simulink model "ALU_Project"  (R2023b)
settings: Solver=VariableStepAuto  StartTime=0.0  StopTime=1  RelTol=1e-3
values from neighbouring files (symbols this model uses):
  A0 = str2num(get(handles.a0i,'string'))    [AluGui.m]
  A1 = str2num(get(handles.a1i,'string'))    [AluGui.m]
  A2 = str2num(get(handles.a2i,'string'))    [AluGui.m]
  A3 = str2num(get(handles.a3i,'string'))    [AluGui.m]
  B0 = str2num(get(handles.b0i,'string'))    [AluGui.m]
  B1 = str2num(get(handles.b1i,'string'))    [AluGui.m]
  B2 = str2num(get(handles.b2i,'string'))    [AluGui.m]
  B3 = str2num(get(handles.b3i,'string'))    [AluGui.m]
  Cin = str2num(get(handles.cii,'string'))    [AluGui.m]
undefined symbols (not defined in the file or in its folder): S0, S1, S2, S3
(part 2 of 2)

== system ALU_Project/15-DECREMENT/HAilf Adder 1 ==
  In1 : Inport
  In2 : Inport  Port=2
  AND : Logic  IconShape=distinctive  AllPortsSameDT=off  OutDataTypeStr=boolean
  XOR : Logic  Operator=XOR  IconShape=distinctive  AllPortsSameDT=off  OutDataTypeStr=boolean
  Sum : Outport
  Carry : Outport  Port=2
  wires:
  In1/1 -> AND/2, XOR/1
  XOR/1 -> Sum/1
  In2/1 -> XOR/2, AND/1
  AND/1 -> Carry/1

== system ALU_Project/15-DECREMENT/HAilf Adder 2 ==
  A1 : Inport
  In2 : Inport  Port=2
  AND : Logic  IconShape=distinctive  AllPortsSameDT=off  OutDataTypeStr=boolean
  XOR : Logic  Operator=XOR  IconShape=distinctive  AllPortsSameDT=off  OutDataTypeStr=boolean
  Sum : Outport
  Carry : Outport  Port=2
  wires:
  A1/1 -> AND/2, XOR/1
  XOR/1 -> Sum/1
  In2/1 -> XOR/2, AND/1
  AND/1 -> Carry/1

== system ALU_Project/15-DECREMENT/HAilf Adder 3 ==
  A2 : Inport
  In2 : Inport  Port=2
  AND : Logic  IconShape=distinctive  AllPortsSameDT=off  OutDataTypeStr=boolean
  XOR : Logic  Operator=XOR  IconShape=distinctive  AllPortsSameDT=off  OutDataTypeStr=boolean
  Sum : Outport
  Carry : Outport  Port=2
  wires:
  A2/1 -> AND/2, XOR/1
  XOR/1 -> Sum/1
  In2/1 -> XOR/2, AND/1
  AND/1 -> Carry/1

== system ALU_Project/15-DECREMENT/HAilf Adder 4 ==
  A3 : Inport
  In2 : Inport  Port=2
  AND : Logic  IconShape=distinctive  AllPortsSameDT=off  OutDataTypeStr=boolean
  XOR : Logic  Operator=XOR  IconShape=distinctive  AllPortsSameDT=off  OutDataTypeStr=boolean
  Sum : Outport
  Carry : Outport  Port=2
  wires:
  A3/1 -> AND/2, XOR/1
  XOR/1 -> Sum/1
  In2/1 -> XOR/2, AND/1
  AND/1 -> Carry/1

== system ALU_Project/15-DECREMENT/HAilf Adder 5 ==
  B0 : Inport
  In2 : Inport  Port=2
  AND : Logic  IconShape=distinctive  AllPortsSameDT=off  OutDataTypeStr=boolean
  XOR : Logic  Operator=XOR  IconShape=distinctive  AllPortsSameDT=off  OutDataTypeStr=boolean
  Sum : Outport
  Carry : Outport  Port=2
  wires:
  B0/1 -> AND/2, XOR/1
  XOR/1 -> Sum/1
  In2/1 -> XOR/2, AND/1
  AND/1 -> Carry/1

== system ALU_Project/15-DECREMENT/HAilf Adder 6 ==
  In1 : Inport
  B1 : Inport  Port=2
  AND : Logic  IconShape=distinctive  AllPortsSameDT=off  OutDataTypeStr=boolean
  XOR : Logic  Operator=XOR  IconShape=distinctive  AllPortsSameDT=off  OutDataTypeStr=boolean
  Sum : Outport
  Carry : Outport  Port=2
  wires:
  In1/1 -> AND/2, XOR/1
  XOR/1 -> Sum/1
  B1/1 -> XOR/2, AND/1
  AND/1 -> Carry/1

== system ALU_Project/15-DECREMENT/HAilf Adder 7 ==
  In1 : Inport
  B2 : Inport  Port=2
  AND : Logic  IconShape=distinctive  AllPortsSameDT=off  OutDataTypeStr=boolean
  XOR : Logic  Operator=XOR  IconShape=distinctive  AllPortsSameDT=off  OutDataTypeStr=boolean
  Sum : Outport
  Carry : Outport  Port=2
  wires:
  In1/1 -> AND/2, XOR/1
  XOR/1 -> Sum/1
  B2/1 -> XOR/2, AND/1
  AND/1 -> Carry/1

== system ALU_Project/15-DECREMENT/HAilf Adder 8 ==
  In1 : Inport
  B3 : Inport  Port=2
  AND : Logic  IconShape=distinctive  AllPortsSameDT=off  OutDataTypeStr=boolean
  XOR : Logic  Operator=XOR  IconShape=distinctive  AllPortsSameDT=off  OutDataTypeStr=boolean
  Sum : Outport
  Carry : Outport  Port=2
  wires:
  In1/1 -> AND/2, XOR/1
  XOR/1 -> Sum/1
  B3/1 -> XOR/2, AND/1
  AND/1 -> Carry/1

== system ALU_Project/16 -Increment/HAilf Adder 1 ==
  In1 : Inport
  In2 : Inport  Port=2
  AND : Logic  IconShape=distinctive  AllPortsSameDT=off  OutDataTypeStr=boolean
  XOR : Logic  Operator=XOR  IconShape=distinctive  AllPortsSameDT=off  OutDataTypeStr=boolean
  Sum : Outport
  Carry : Outport  Port=2
  wires:
  In1/1 -> AND/2, XOR/1
  XOR/1 -> Sum/1
  In2/1 -> XOR/2, AND/1
  AND/1 -> Carry/1

== system ALU_Project/16 -Increment/HAilf Adder 2 ==
  A1 : Inport
  In2 : Inport  Port=2
  AND : Logic  IconShape=distinctive  AllPortsSameDT=off  OutDataTypeStr=boolean
  XOR : Logic  Operator=XOR  IconShape=distinctive  AllPortsSameDT=off  OutDataTypeStr=boolean
  Sum : Outport
  Carry : Outport  Port=2
  wires:
  A1/1 -> AND/2, XOR/1
  XOR/1 -> Sum/1
  In2/1 -> XOR/2, AND/1
  AND/1 -> Carry/1

== system ALU_Project/16 -Increment/HAilf Adder 3 ==
  A2 : Inport
  In2 : Inport  Port=2
  AND : Logic  IconShape=distinctive  AllPortsSameDT=off  OutDataTypeStr=boolean
  XOR : Logic  Operator=XOR  IconShape=distinctive  AllPortsSameDT=off  OutDataTypeStr=boolean
  Sum : Outport
  Carry : Outport  Port=2
  wires:
  A2/1 -> AND/2, XOR/1
  XOR/1 -> Sum/1
  In2/1 -> XOR/2, AND/1
  AND/1 -> Carry/1

== system ALU_Project/16 -Increment/HAilf Adder 4 ==
  A3 : Inport
  In2 : Inport  Port=2
  AND : Logic  IconShape=distinctive  AllPortsSameDT=off  OutDataTypeStr=boolean
  XOR : Logic  Operator=XOR  IconShape=distinctive  AllPortsSameDT=off  OutDataTypeStr=boolean
  Sum : Outport
  Carry : Outport  Port=2
  wires:
  A3/1 -> AND/2, XOR/1
  XOR/1 -> Sum/1
  In2/1 -> XOR/2, AND/1
  AND/1 -> Carry/1

== system ALU_Project/16 -Increment/HAilf Adder 5 ==
  B0 : Inport
  In2 : Inport  Port=2
  AND : Logic  IconShape=distinctive  AllPortsSameDT=off  OutDataTypeStr=boolean
  XOR : Logic  Operator=XOR  IconShape=distinctive  AllPortsSameDT=off  OutDataTypeStr=boolean
  Sum : Outport
  Carry : Outport  Port=2
  wires:
  B0/1 -> AND/2, XOR/1
  XOR/1 -> Sum/1
  In2/1 -> XOR/2, AND/1
  AND/1 -> Carry/1

== system ALU_Project/16 -Increment/HAilf Adder 6 ==
  In1 : Inport
  B1 : Inport  Port=2
  AND : Logic  IconShape=distinctive  AllPortsSameDT=off  OutDataTypeStr=boolean
  XOR : Logic  Operator=XOR  IconShape=distinctive  AllPortsSameDT=off  OutDataTypeStr=boolean
  Sum : Outport
  Carry : Outport  Port=2
  wires:
  In1/1 -> AND/2, XOR/1
  XOR/1 -> Sum/1
  B1/1 -> XOR/2, AND/1
  AND/1 -> Carry/1

== system ALU_Project/16 -Increment/HAilf Adder 7 ==
  In1 : Inport
  B2 : Inport  Port=2
  AND : Logic  IconShape=distinctive  AllPortsSameDT=off  OutDataTypeStr=boolean
  XOR : Logic  Operator=XOR  IconShape=distinctive  AllPortsSameDT=off  OutDataTypeStr=boolean
  Sum : Outport
  Carry : Outport  Port=2
  wires:
  In1/1 -> AND/2, XOR/1
  XOR/1 -> Sum/1
  B2/1 -> XOR/2, AND/1
  AND/1 -> Carry/1

== system ALU_Project/16 -Increment/HAilf Adder 8 ==
  In1 : Inport
  B3 : Inport  Port=2
  AND : Logic  IconShape=distinctive  AllPortsSameDT=off  OutDataTypeStr=boolean
  XOR : Logic  Operator=XOR  IconShape=distinctive  AllPortsSameDT=off  OutDataTypeStr=boolean
  Sum : Outport
  Carry : Outport  Port=2
  wires:
  In1/1 -> AND/2, XOR/1
  XOR/1 -> Sum/1
  B3/1 -> XOR/2, AND/1
  AND/1 -> Carry/1
